simulink model "RW_1_testmode"  (R2018a)
settings: Solver=ode4  StartTime=0  StopTime=1000  FixedStep=ConfParam.confOrbit.dt  RelTol=1e-3
undefined symbols (not defined in the file): ConfParam, import_orbit, RWS, Subsystem
libraries: ComputeNorm3D x5, simulink x4, sharedtransform x2, Command x1, Date x1, KepOrbit x1, Estimator x1, BdotController x1, RWS_1W_PDcontroller x1, IGRF x1, SunEphemeris_MathWorks x1, MTB x1
settings Model: Creator=Cédric  LastModifiedBy=Cédric
settings DataIOCC: SaveTime=off
settings DebuggingCC: MultiTaskRateTransMsg=warning

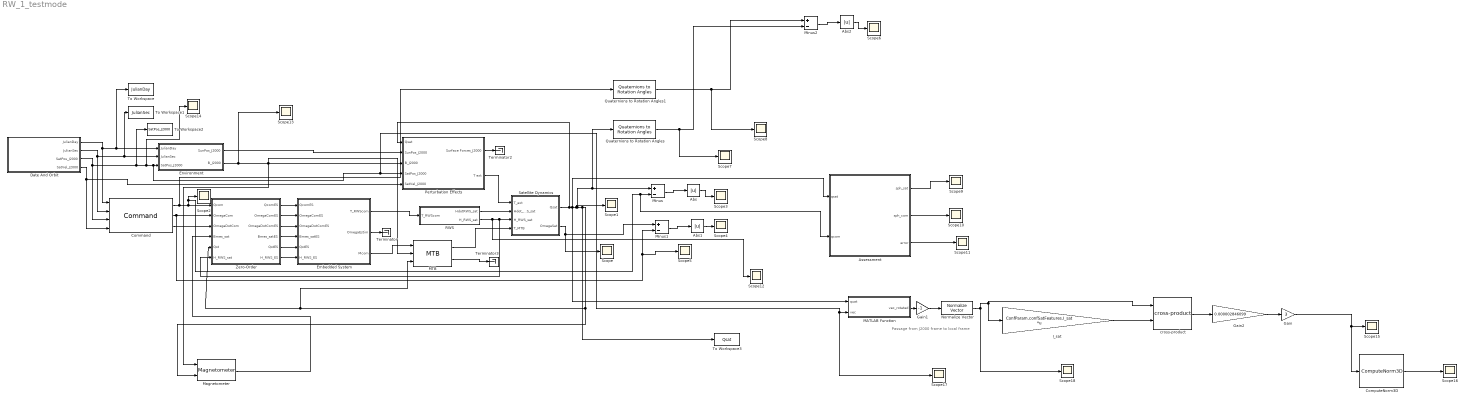
== system RW_1_testmode ==
  note: Passage from J2000 frame to local frame
  Abs : Abs
  Abs1 : Abs
  Abs2 : Abs
  Assessment : Subsystem
  Command : Command/Command
  ComputeNorm3D : ComputeNorm3D/ComputeNorm3D
  Date And Orbit : Subsystem
  Embedded System : Subsystem
  Environment : Subsystem
  Gain : Gain  Gain=3
  Gain1 : Gain  Gain=-1
  Gain2 : Gain  Gain=0.000002846099
  I_sat : Gain  Gain=ConfParam.confSatFeatures.I_sat  Multiplication=Matrix(K*u)
  MATLAB Function : MATLAB Function  TreatAsAtomicUnit=on
  MTB : MTB/MTB
  Magnetometer : Magnetometer/Magnetometer
  Minus : Sum  Inputs=+-
  Minus1 : Sum  Inputs=+-
  Minus2 : Sum  Inputs=+-
  Normalize Vector : vrlib/Utilities/Normalize Vector  maxzero=0
      settings: SourceProductName=Simulink 3D Animation  SourceProductBaseCode=VR
  Perturbation Effects : Subsystem
  Quaternions to Rotation Angles : sharedtransform/Quaternions to Rotation Angles  rotationOrder=ZYX  aMode=aMode
      settings: SourceProductBaseCode=AE
  Quaternions to Rotation Angles1 : sharedtransform/Quaternions to Rotation Angles  rotationOrder=ZYX  aMode=aMode
      settings: SourceProductBaseCode=AE
  RWS : Subsystem  AncestorBlock=RWS/RWS
  Satellite Dynamics : Subsystem  AncestorBlock=SatDyn/Satellite Dynamics
  Scope{,1..18} (19 alike) : Scope
  Terminator : Terminator
  Terminator2 : Terminator
  Terminator3 : Terminator
  To Workspace : ToWorkspace  VariableName=JulianDay  SampleTime=-1
  To Workspace1 : ToWorkspace  VariableName=JulianSec  SampleTime=-1
  To Workspace2 : ToWorkspace  VariableName=SatPos_J2000  SampleTime=-1
  To Workspace3 : ToWorkspace  VariableName=Qsat  SampleTime=-1
  Zero-Order : Subsystem
  cross-product : CrossProd/cross-product
  wires:
  Date And Orbit/1(JulianDay) -> To Workspace/1, Environment/1(JulianDay), Command/1
  Date And Orbit/2(JulianSec) -> To Workspace1/1, Environment/2(JulianSec), Command/2
  Date And Orbit/3(SatPos_J2000) -> To Workspace2/1, Scope14/1, Scope17/1, MATLAB Function/2(vec), Perturbation Effects/4(SatPos_J2000), Environment/3(SatPos_J2000), Command/3
  Date And Orbit/4(SatVel_J2000) -> Perturbation Effects/5(SatVel_J2000), Command/4
  Environment/1(SunPos_J2000) -> Perturbation Effects/2(SunPos_J2000)
  Environment/2(B_J2000) -> Scope13/1, Perturbation Effects/3(B_J2000), Magnetometer/1, MTB/2
  Command/1 -> Quaternions to Rotation Angles1/1, Assessment/2(qcom), Minus/2, Scope2/1, Zero-Order/1(Qcom)
  Command/2 -> Scope5/1, Minus1/2, Zero-Order/2(OmegaCom)
  Command/3 -> Zero-Order/3(OmegaDotCom)
  Zero-Order/1(QcomES) -> Embedded System/1(QcomES)
  Zero-Order/2(OmegaComES) -> Embedded System/2(OmegaComES)
  Zero-Order/3(OmegaDotComES) -> Embedded System/3(OmegaDotComES)
  Zero-Order/4(Bmes_satES) -> Embedded System/4(Bmes_satES)
  Zero-Order/5(QstES) -> Embedded System/5(QstES)
  Zero-Order/6(H_RWS_ES) -> Embedded System/6(H_RWS_ES)
  Embedded System/3(Mcom) -> MTB/1
  MTB/1 -> Satellite Dynamics/4(T_MTB)
  Magnetometer/1 -> Zero-Order/4(Bmes_sat)
  Embedded System/2(OmegaEstim) -> Terminator/1
  Satellite Dynamics/2(OmegaSat) -> Minus1/1, Scope/1
  Perturbation Effects/1(Surface Forces_J2000) -> Terminator2/1
  Minus/1 -> Abs/1
  Abs/1 -> Scope3/1
  Minus1/1 -> Abs1/1
  Abs1/1 -> Scope4/1
  Abs2/1 -> Scope6/1
  Minus2/1 -> Abs2/1
  Quaternions to Rotation Angles1/1 -> Scope8/1, Minus2/1
  Quaternions to Rotation Angles/1 -> Scope7/1, Minus2/2
  MTB/2 -> Terminator3/1
  RWS/2(H_RWS_sat) -> Scope12/1, Satellite Dynamics/3(H_RWS_sat), Zero-Order/6(H_RWS_sat)
  Embedded System/1(T_RWScom) -> RWS/1(T_RWScom)
  Perturbation Effects/2(T ext) -> Satellite Dynamics/1(T_ext)
  RWS/1(HdotRWS_sat) -> Satellite Dynamics/2(Hdot_RWS_sat)
  Gain2/1 -> Gain/1
  Gain/1 -> ComputeNorm3D/1, Scope15/1
  cross-product/1 -> Gain2/1
  I_sat/1 -> cross-product/2
  MATLAB Function/1(vec_rotated) -> Gain1/1
  ComputeNorm3D/1 -> Scope16/1
  Assessment/3(error) -> Scope11/1
  Assessment/2(sph_com) -> Scope10/1
  Assessment/1(sph_sat) -> Scope9/1
  Satellite Dynamics/1(Qsat) -> Perturbation Effects/1(Qsat), MATLAB Function/1(quat), Assessment/1(qsat), Scope1/1, Quaternions to Rotation Angles/1, Minus/1, To Workspace3/1, MTB/3, Zero-Order/5(Qst), Magnetometer/2
  Gain1/1 -> Normalize Vector/1
  Normalize Vector/1 -> I_sat/1, cross-product/1, Scope18/1

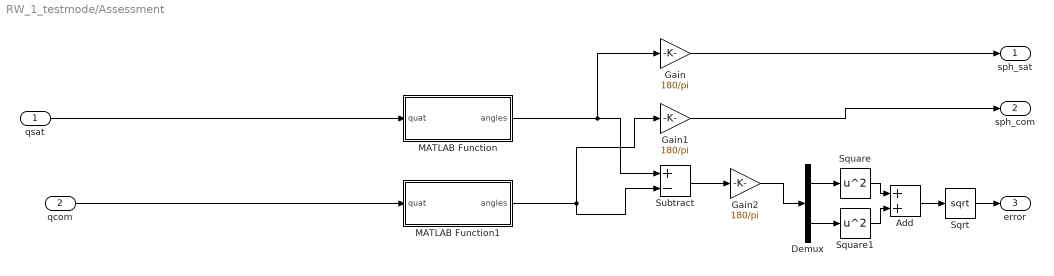
== system RW_1_testmode/Assessment ==
  qsat : Inport
  qcom : Inport  Port=2
  Add : Sum
  Demux : Demux  Outputs=2
  Gain : Gain  Gain=180/pi
  Gain1 : Gain  Gain=180/pi
  Gain2 : Gain  Gain=180/pi
  MATLAB Function : MATLAB Function  TreatAsAtomicUnit=on
  MATLAB Function1 : MATLAB Function  TreatAsAtomicUnit=on
  Sqrt : Sqrt  SaturateOnIntegerOverflow=on
  Square : Math  Operator=square  SaturateOnIntegerOverflow=on
  Square1 : Math  Operator=square  SaturateOnIntegerOverflow=on
  Subtract : Sum  Inputs=+-
  sph_sat : Outport
  sph_com : Outport  Port=2
  error : Outport  Port=3
  wires:
  MATLAB Function1/1(angles) -> Subtract/2, Gain1/1
  MATLAB Function/1(angles) -> Gain/1, Subtract/1
  Subtract/1 -> Gain2/1
  qsat/1 -> MATLAB Function/1(quat)
  Gain/1 -> sph_sat/1
  Gain1/1 -> sph_com/1
  Gain2/1 -> Demux/1
  Demux/1 -> Square/1
  Demux/2 -> Square1/1
  Square/1 -> Add/1
  Square1/1 -> Add/2
  Add/1 -> Sqrt/1
  Sqrt/1 -> error/1
  qcom/1 -> MATLAB Function1/1(quat)

== system RW_1_testmode/Date And Orbit ==
  Clock : Clock
  Current Simulation Date : Date/Current Simulation Date
  Orbit : KepOrbit/Keplerian Orbit
  Pierre's orbit : Subsystem  Commented=on  AncestorBlock=import_orbit/Subsystem
  JulianDay : Outport
  JulianSec : Outport  Port=2
  SatPos_J2000 : Outport  Port=3
  SatVel_J2000 : Outport  Port=4
  wires:
  Current Simulation Date/1 -> JulianDay/1
  Current Simulation Date/2 -> JulianSec/1
  Clock/1 -> Current Simulation Date/1
  Orbit/2 -> SatVel_J2000/1
  Orbit/1 -> SatPos_J2000/1

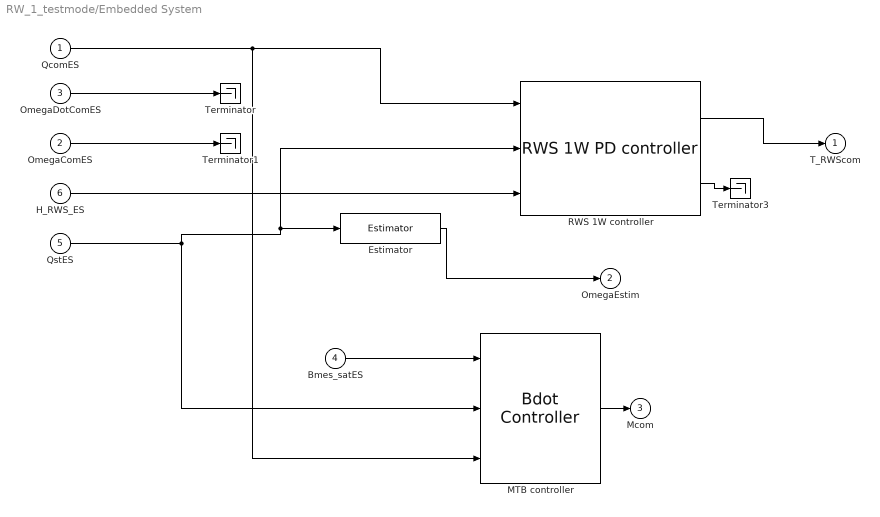
== system RW_1_testmode/Embedded System ==
  QcomES : Inport
  OmegaComES : Inport  Port=2
  OmegaDotComES : Inport  Port=3
  Bmes_satES : Inport  Port=4
  QstES : Inport  Port=5
  H_RWS_ES : Inport  Port=6
  Estimator : Estimator/Estimator
  MTB controller : BdotController/Bdot Controller
  RWS 1W controller : RWS_1W_PDcontroller/RWS 1W PD controller
  Terminator : Terminator
  Terminator1 : Terminator
  Terminator3 : Terminator
  T_RWScom : Outport
  OmegaEstim : Outport  Port=2
  Mcom : Outport  Port=3
  wires:
  QstES/1 -> MTB controller/2, RWS 1W controller/2, Estimator/1
  Estimator/1 -> OmegaEstim/1
  Bmes_satES/1 -> MTB controller/1
  MTB controller/1 -> Mcom/1
  QcomES/1 -> MTB controller/3, RWS 1W controller/1
  H_RWS_ES/1 -> RWS 1W controller/3
  OmegaComES/1 -> Terminator1/1
  OmegaDotComES/1 -> Terminator/1
  RWS 1W controller/1 -> T_RWScom/1
  RWS 1W controller/2 -> Terminator3/1

== system RW_1_testmode/Environment ==
  JulianDay : Inport
  JulianSec : Inport  Port=2
  SatPos_J2000 : Inport  Port=3
  B J2000 : IGRF/IGRF in the J2000 frame
  Sun Ephemeris J2000 : SunEphemeris_MathWorks/Sun Ephemeris J2000
  SunPos_J2000 : Outport
  B_J2000 : Outport  Port=2
  wires:
  Sun Ephemeris J2000/1 -> SunPos_J2000/1
  JulianDay/1 -> Sun Ephemeris J2000/1, B J2000/1
  JulianSec/1 -> Sun Ephemeris J2000/2, B J2000/2
  SatPos_J2000/1 -> B J2000/3
  B J2000/1 -> B_J2000/1

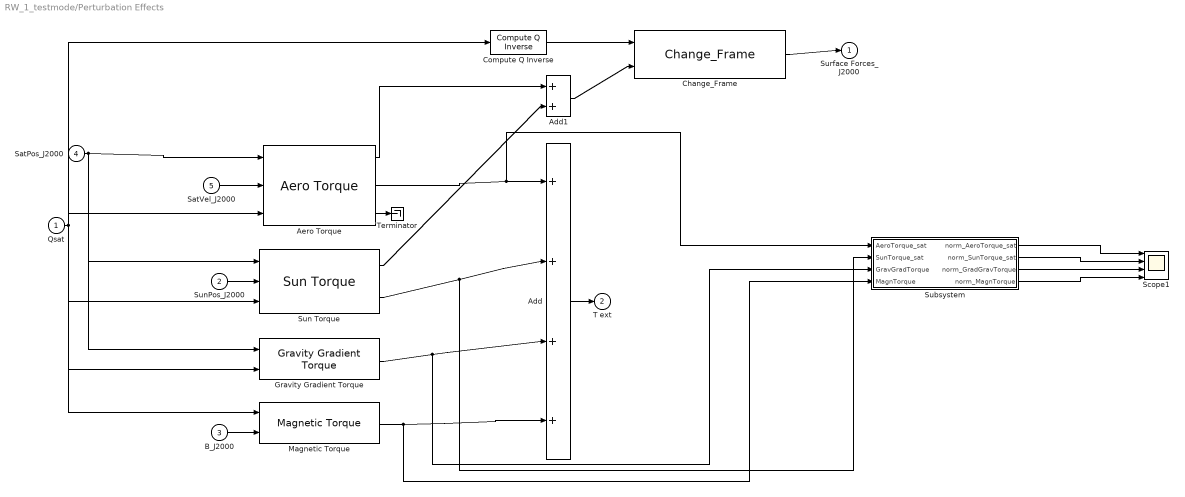
== system RW_1_testmode/Perturbation Effects ==
  Qsat : Inport
  SunPos_J2000 : Inport  Port=2
  B_J2000 : Inport  Port=3
  SatPos_J2000 : Inport  Port=4
  SatVel_J2000 : Inport  Port=5
  Add : Sum  Inputs=++++
  Add1 : Sum
  Aero Torque : AeroTorqueA/Aero Torque
  Change_Frame : ChangeFrame/Change_Frame
  Compute Q Inverse : Qinverse/Compute Q Inverse
  Gravity Gradient Torque : GravGradTorque/Gravity Gradient Torque
  Magnetic Torque : MagnTorque/Magnetic Torque
  Scope1 : Scope  NumInputPorts=4
  Subsystem : Subsystem
  Sun Torque : SunTorqueA/Sun Torque
  Terminator : Terminator
  Surface Forces_J2000 : Outport
  T ext : Outport  Port=2
  wires:
  Compute Q Inverse/1 -> Change_Frame/1
  Change_Frame/1 -> Surface Forces_J2000/1
  Qsat/1 -> Compute Q Inverse/1, Gravity Gradient Torque/2, Sun Torque/3, Magnetic Torque/1, Aero Torque/3
  SunPos_J2000/1 -> Sun Torque/2
  B_J2000/1 -> Magnetic Torque/2
  SatPos_J2000/1 -> Sun Torque/1, Gravity Gradient Torque/1, Aero Torque/1
  SatVel_J2000/1 -> Aero Torque/2
  Aero Torque/3 -> Terminator/1
  Add1/1 -> Change_Frame/2
  Aero Torque/1 -> Add1/1
  Sun Torque/1 -> Add1/2
  Add/1 -> T ext/1
  Aero Torque/2 -> Subsystem/1(AeroTorque_sat), Add/1
  Sun Torque/2 -> Subsystem/2(SunTorque_sat), Add/2
  Gravity Gradient Torque/1 -> Subsystem/3(GravGradTorque), Add/3
  Magnetic Torque/1 -> Subsystem/4(MagnTorque), Add/4
  Subsystem/1(norm_AeroTorque_sat) -> Scope1/1
  Subsystem/2(norm_SunTorque_sat) -> Scope1/2
  Subsystem/3(norm_GradGravTorque) -> Scope1/3
  Subsystem/4(norm_MagnTorque) -> Scope1/4

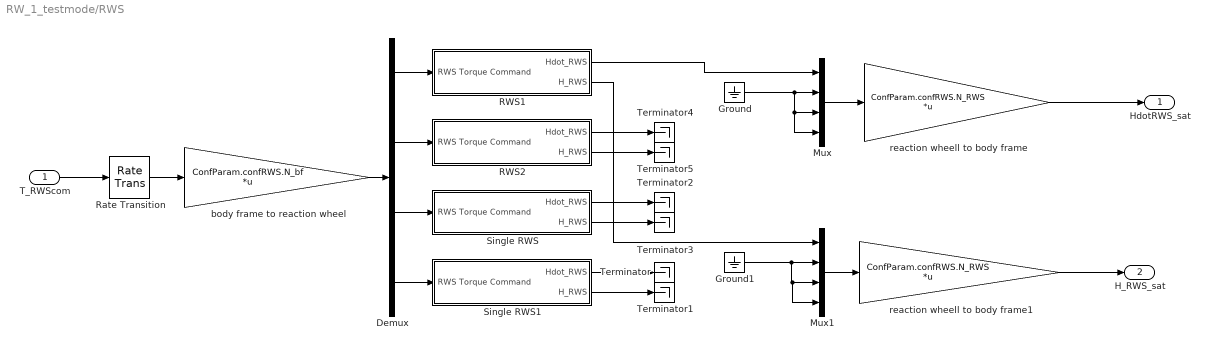
== system RW_1_testmode/RWS ==
  T_RWScom : Inport
  Demux : Demux
  Ground : Ground
  Ground1 : Ground
  Mux : Mux
  Mux1 : Mux
  RWS1 : Subsystem  AncestorBlock=SingleRWS/Single RWS
  RWS2 : Subsystem
  Rate Transition : RateTransition  InitialCondition=[0;0;0]  OutPortSampleTime=ConfParam.confOrbit.dt
  Single RWS : Subsystem
  Single RWS1 : Subsystem
  Terminator{,1..5} (6 alike) : Terminator
  body frame to reaction wheel : Gain  Gain=ConfParam.confRWS.N_bf  Multiplication=Matrix(K*u)
  reaction wheell to body frame : Gain  Gain=ConfParam.confRWS.N_RWS  Multiplication=Matrix(K*u)
  reaction wheell to body frame1 : Gain  Gain=ConfParam.confRWS.N_RWS  Multiplication=Matrix(K*u)
  HdotRWS_sat : Outport
  H_RWS_sat : Outport  Port=2
  wires:
  Ground1/1 -> Mux1/2, Mux1/3, Mux1/4
  Ground/1 -> Mux/2, Mux/3, Mux/4
  RWS2/2(H_RWS) -> Terminator5/1
  RWS2/1(Hdot_RWS) -> Terminator4/1
  Single RWS/2(H_RWS) -> Terminator3/1
  Single RWS/1(Hdot_RWS) -> Terminator2/1
  Single RWS1/2(H_RWS) -> Terminator1/1
  Single RWS1/1(Hdot_RWS) -> Terminator/1
  Mux1/1 -> reaction wheell to body frame1/1
  Demux/2 -> RWS2/1(RWS Torque Command)
  Demux/4 -> Single RWS1/1(RWS Torque Command)
  Demux/3 -> Single RWS/1(RWS Torque Command)
  RWS1/1(Hdot_RWS) -> Mux/1
  reaction wheell to body frame/1 -> HdotRWS_sat/1
  reaction wheell to body frame1/1 -> H_RWS_sat/1
  RWS1/2(H_RWS) -> Mux1/1
  Mux/1 -> reaction wheell to body frame/1
  Demux/1 -> RWS1/1(RWS Torque Command)
  body frame to reaction wheel/1 -> Demux/1
  T_RWScom/1 -> Rate Transition/1
  Rate Transition/1 -> body frame to reaction wheel/1

== system RW_1_testmode/Satellite Dynamics ==
  T_ext : Inport
  Hdot_RWS_sat : Inport  Port=2
  H_RWS_sat : Inport  Port=3
  T_MTB : Inport  Port=4
  Compute Omega Sat : Subsystem
  Constant : Constant  Value=0
  Gain : Gain  Gain=1/2
  Integrator : Integrator  InitialCondition=ConfParam.confSatDyn.InitQsat
  Mux : Mux  Inputs=2
  QuatProd : Subsystem  TreatAsAtomicUnit=on
      settings: RTWFcnNameOpts=Use subsystem name  RTWFileNameOpts=Use subsystem name
  Qsat : Outport
  OmegaSat : Outport  Port=2
  wires:
  H_RWS_sat/1 -> Compute Omega Sat/3(H_RWS_sat)
  QuatProd/1("q\"") -> Gain/1
  T_MTB/1 -> Compute Omega Sat/4(T_MTB)
  Constant/1 -> Mux/1
  Hdot_RWS_sat/1 -> Compute Omega Sat/2(Hdot_RWS_sat)
  Gain/1 -> Integrator/1
  Integrator/1 -> QuatProd/1(q), Qsat/1
  Mux/1 -> QuatProd/2(q')
  Compute Omega Sat/1(OmegaSat) -> Mux/2, OmegaSat/1
  T_ext/1 -> Compute Omega Sat/1(T_ext)

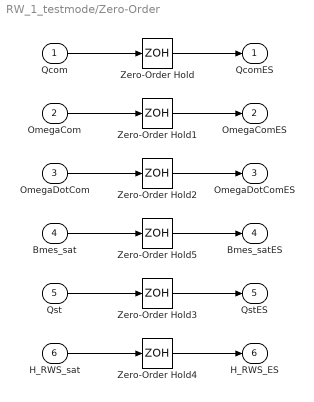
== system RW_1_testmode/Zero-Order ==
  Qcom : Inport
  OmegaCom : Inport  Port=2
  OmegaDotCom : Inport  Port=3
  Bmes_sat : Inport  Port=4
  Qst : Inport  Port=5
  H_RWS_sat : Inport  Port=6
  Zero-Order Hold{,1..5} (6 alike) : ZeroOrderHold  SampleTime=1/ConfParam.confES.frequency
  QcomES : Outport
  OmegaComES : Outport  Port=2
  OmegaDotComES : Outport  Port=3
  Bmes_satES : Outport  Port=4
  QstES : Outport  Port=5
  H_RWS_ES : Outport  Port=6
  wires:
  Qcom/1 -> Zero-Order Hold/1
  Zero-Order Hold/1 -> QcomES/1
  OmegaCom/1 -> Zero-Order Hold1/1
  Zero-Order Hold1/1 -> OmegaComES/1
  OmegaDotCom/1 -> Zero-Order Hold2/1
  Zero-Order Hold2/1 -> OmegaDotComES/1
  Qst/1 -> Zero-Order Hold3/1
  Zero-Order Hold3/1 -> QstES/1
  H_RWS_sat/1 -> Zero-Order Hold4/1
  Zero-Order Hold4/1 -> H_RWS_ES/1
  Bmes_sat/1 -> Zero-Order Hold5/1
  Zero-Order Hold5/1 -> Bmes_satES/1

== system RW_1_testmode/Date And Orbit/Pierre's orbit ==
  Demux : Demux  Outputs=6
  From File : FromFile  FileName=C:\Users\cedri\Documents\TOLOSAT\tolosat_adcs\pythondev\positions\timestamped_file.mat  SampleTime=1  ExtrapolationBeforeFirstDataPoint=Hold first value  InterpolationWithinTimeRange=Zero order hold  ExtrapolationAfterLastDataPoint=Hold last value
  Mux : Mux  Inputs=3
  Mux1 : Mux  Inputs=3
  Positions : Scope
  Velocities : Scope
  SatVel_J2000 : Outport
  SatPos_J2000 : Outport  Port=2
  wires:
  Demux/6 -> Mux1/3
  Mux1/1 -> Positions/1, SatPos_J2000/1
  Demux/4 -> Mux1/1
  From File/1 -> Demux/1
  Mux/1 -> Velocities/1, SatVel_J2000/1
  Demux/1 -> Mux/1
  Demux/2 -> Mux/2
  Demux/3 -> Mux/3
  Demux/5 -> Mux1/2

== system RW_1_testmode/Perturbation Effects/Subsystem ==
  AeroTorque_sat : Inport
  SunTorque_sat : Inport  Port=2
  GravGradTorque : Inport  Port=3
  MagnTorque : Inport  Port=4
  ComputeNorm3D{,1..3} (4 alike) : ComputeNorm3D/ComputeNorm3D
  norm_AeroTorque_sat : Outport
  norm_SunTorque_sat : Outport  Port=2
  norm_GradGravTorque : Outport  Port=3
  norm_MagnTorque : Outport  Port=4
  wires:
  GravGradTorque/1 -> ComputeNorm3D1/1
  ComputeNorm3D1/1 -> norm_GradGravTorque/1
  AeroTorque_sat/1 -> ComputeNorm3D/1
  MagnTorque/1 -> ComputeNorm3D3/1
  ComputeNorm3D2/1 -> norm_SunTorque_sat/1
  SunTorque_sat/1 -> ComputeNorm3D2/1
  ComputeNorm3D3/1 -> norm_MagnTorque/1
  ComputeNorm3D/1 -> norm_AeroTorque_sat/1

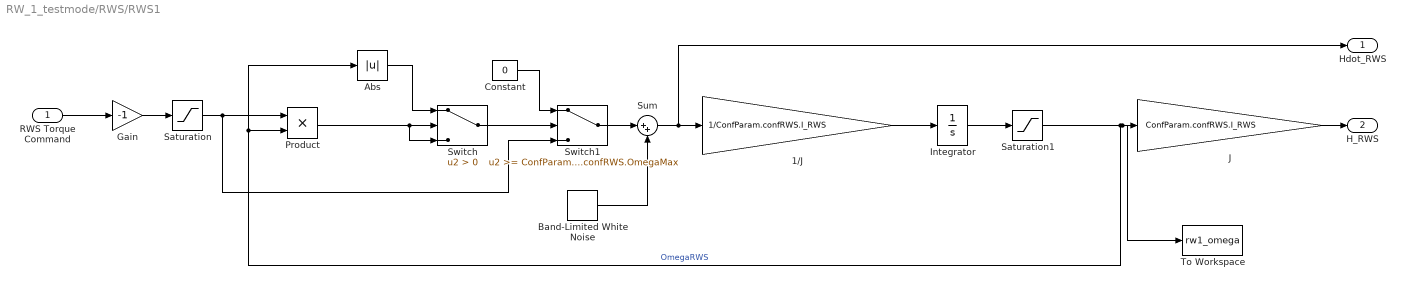
== system RW_1_testmode/RWS/RWS1 ==
  RWS Torque Command : Inport
  1/J : Gain  Gain=1/ConfParam.confRWS.I_RWS
  Abs : Abs
  Band-Limited White Noise : simulink/Sources/Band-Limited White Noise  Cov=ConfParam.confRWS.NoisePower  Ts=ConfParam.confOrbit.dt  seed=[23341]
  Constant : Constant  Value=0
  Gain : Gain  Gain=-1
  Integrator : Integrator  InitialCondition=ConfParam.confRWS.IntitOmegaRWS(1)
  J : Gain  Gain=ConfParam.confRWS.I_RWS
  Product : Product
  Saturation : Saturate  UpperLimit=ConfParam.confRWS.Tmax  LowerLimit=-ConfParam.confRWS.Tmax
  Saturation1 : Saturate  UpperLimit=ConfParam.confRWS.OmegaMax  LowerLimit=-ConfParam.confRWS.OmegaMax
  Sum : Sum  Inputs=|++
  Switch : Switch  Criteria=u2 > Threshold
  Switch1 : Switch  Threshold=ConfParam.confRWS.OmegaMax
  To Workspace : ToWorkspace  VariableName=rw1_omega  SampleTime=-1
  Hdot_RWS : Outport
  H_RWS : Outport  Port=2
  wires:
  Switch1/1 -> Sum/1
  Switch/1 -> Switch1/2
  Constant/1 -> Switch1/1
  RWS Torque Command/1 -> Gain/1
  Product/1 -> Switch/2, Switch/3
  Saturation/1 -> Product/1, Switch1/3
  Integrator/1 -> Saturation1/1
  Saturation1/1 -> To Workspace/1, J/1, Abs/1, Product/2  "OmegaRWS"
  Sum/1 -> Hdot_RWS/1, 1/J/1
  1/J/1 -> Integrator/1
  Abs/1 -> Switch/1
  J/1 -> H_RWS/1
  Band-Limited White Noise/1 -> Sum/2
  Gain/1 -> Saturation/1

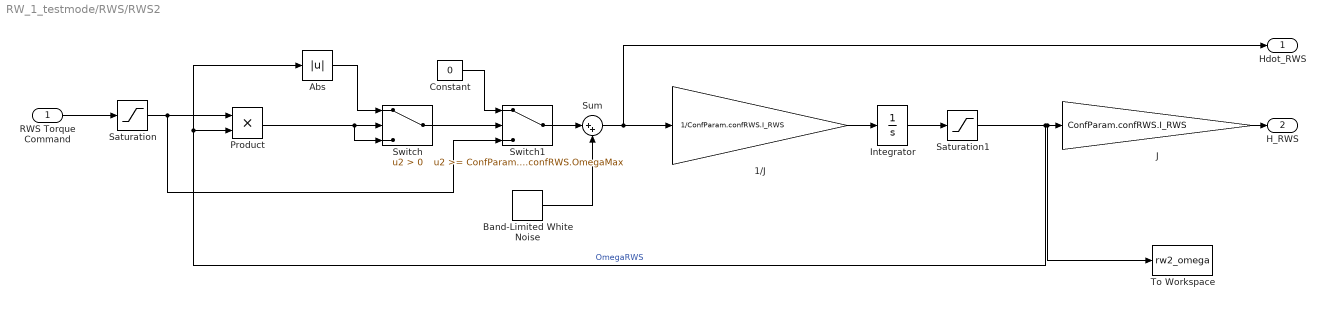
== system RW_1_testmode/RWS/RWS2 ==
  RWS Torque Command : Inport
  1/J : Gain  Gain=1/ConfParam.confRWS.I_RWS
  Abs : Abs
  Band-Limited White Noise : simulink/Sources/Band-Limited White Noise  Cov=ConfParam.confRWS.NoisePower  Ts=ConfParam.confOrbit.dt  seed=[23341]
  Constant : Constant  Value=0
  Integrator : Integrator  InitialCondition=ConfParam.confRWS.IntitOmegaRWS(2)
  J : Gain  Gain=ConfParam.confRWS.I_RWS
  Product : Product
  Saturation : Saturate  UpperLimit=ConfParam.confRWS.Tmax  LowerLimit=-ConfParam.confRWS.Tmax
  Saturation1 : Saturate  UpperLimit=ConfParam.confRWS.OmegaMax  LowerLimit=-ConfParam.confRWS.OmegaMax
  Sum : Sum  Inputs=|++
  Switch : Switch  Criteria=u2 > Threshold
  Switch1 : Switch  Threshold=ConfParam.confRWS.OmegaMax
  To Workspace : ToWorkspace  VariableName=rw2_omega  SampleTime=-1
  Hdot_RWS : Outport
  H_RWS : Outport  Port=2
  wires:
  Switch1/1 -> Sum/1
  Switch/1 -> Switch1/2
  Constant/1 -> Switch1/1
  RWS Torque Command/1 -> Saturation/1
  Product/1 -> Switch/2, Switch/3
  Saturation/1 -> Product/1, Switch1/3
  Integrator/1 -> Saturation1/1
  Saturation1/1 -> Abs/1, Product/2, To Workspace/1, J/1  "OmegaRWS"
  Sum/1 -> Hdot_RWS/1, 1/J/1
  1/J/1 -> Integrator/1
  Abs/1 -> Switch/1
  J/1 -> H_RWS/1
  Band-Limited White Noise/1 -> Sum/2

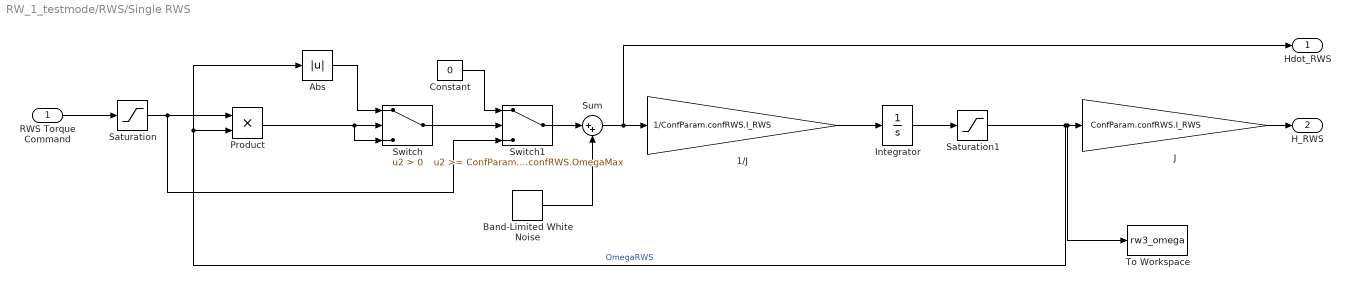
== system RW_1_testmode/RWS/Single RWS ==
  RWS Torque Command : Inport
  1/J : Gain  Gain=1/ConfParam.confRWS.I_RWS
  Abs : Abs
  Band-Limited White Noise : simulink/Sources/Band-Limited White Noise  Cov=ConfParam.confRWS.NoisePower  Ts=ConfParam.confOrbit.dt  seed=[23341]
  Constant : Constant  Value=0
  Integrator : Integrator  InitialCondition=ConfParam.confRWS.IntitOmegaRWS(3)
  J : Gain  Gain=ConfParam.confRWS.I_RWS
  Product : Product
  Saturation : Saturate  UpperLimit=ConfParam.confRWS.Tmax  LowerLimit=-ConfParam.confRWS.Tmax
  Saturation1 : Saturate  UpperLimit=ConfParam.confRWS.OmegaMax  LowerLimit=-ConfParam.confRWS.OmegaMax
  Sum : Sum  Inputs=|++
  Switch : Switch  Criteria=u2 > Threshold
  Switch1 : Switch  Threshold=ConfParam.confRWS.OmegaMax
  To Workspace : ToWorkspace  VariableName=rw3_omega  SampleTime=-1
  Hdot_RWS : Outport
  H_RWS : Outport  Port=2
  wires:
  Switch1/1 -> Sum/1
  Switch/1 -> Switch1/2
  Constant/1 -> Switch1/1
  RWS Torque Command/1 -> Saturation/1
  Product/1 -> Switch/2, Switch/3
  Saturation/1 -> Product/1, Switch1/3
  Integrator/1 -> Saturation1/1
  Saturation1/1 -> To Workspace/1, J/1, Abs/1, Product/2  "OmegaRWS"
  Sum/1 -> Hdot_RWS/1, 1/J/1
  1/J/1 -> Integrator/1
  Abs/1 -> Switch/1
  J/1 -> H_RWS/1
  Band-Limited White Noise/1 -> Sum/2

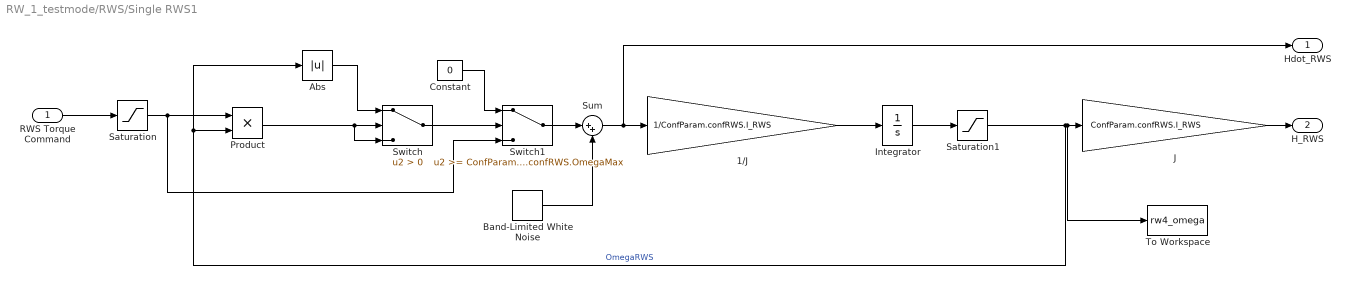
== system RW_1_testmode/RWS/Single RWS1 ==
  RWS Torque Command : Inport
  1/J : Gain  Gain=1/ConfParam.confRWS.I_RWS
  Abs : Abs
  Band-Limited White Noise : simulink/Sources/Band-Limited White Noise  Cov=ConfParam.confRWS.NoisePower  Ts=ConfParam.confOrbit.dt  seed=[23341]
  Constant : Constant  Value=0
  Integrator : Integrator  InitialCondition=ConfParam.confRWS.IntitOmegaRWS(4)
  J : Gain  Gain=ConfParam.confRWS.I_RWS
  Product : Product
  Saturation : Saturate  UpperLimit=ConfParam.confRWS.Tmax  LowerLimit=-ConfParam.confRWS.Tmax
  Saturation1 : Saturate  UpperLimit=ConfParam.confRWS.OmegaMax  LowerLimit=-ConfParam.confRWS.OmegaMax
  Sum : Sum  Inputs=|++
  Switch : Switch  Criteria=u2 > Threshold
  Switch1 : Switch  Threshold=ConfParam.confRWS.OmegaMax
  To Workspace : ToWorkspace  VariableName=rw4_omega  SampleTime=-1
  Hdot_RWS : Outport
  H_RWS : Outport  Port=2
  wires:
  Switch1/1 -> Sum/1
  Switch/1 -> Switch1/2
  Constant/1 -> Switch1/1
  RWS Torque Command/1 -> Saturation/1
  Product/1 -> Switch/2, Switch/3
  Saturation/1 -> Product/1, Switch1/3
  Integrator/1 -> Saturation1/1
  Saturation1/1 -> To Workspace/1, J/1, Abs/1, Product/2  "OmegaRWS"
  Sum/1 -> Hdot_RWS/1, 1/J/1
  1/J/1 -> Integrator/1
  Abs/1 -> Switch/1
  J/1 -> H_RWS/1
  Band-Limited White Noise/1 -> Sum/2

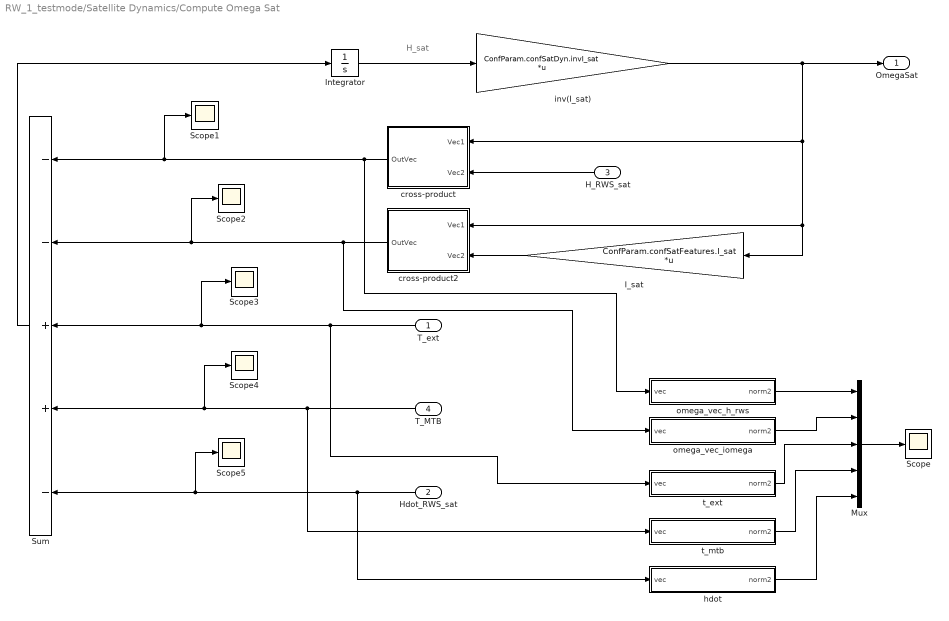
== system RW_1_testmode/Satellite Dynamics/Compute Omega Sat ==
  note: H_sat
  T_ext : Inport
  Hdot_RWS_sat : Inport  Port=2
  H_RWS_sat : Inport  Port=3
  T_MTB : Inport  Port=4
  I_sat : Gain  Gain=ConfParam.confSatFeatures.I_sat  Multiplication=Matrix(K*u)
  Integrator : Integrator  InitialCondition=ConfParam.confSatFeatures.I_sat*ConfParam.confSatDyn.InitOmega_sat
  Mux : Mux  Inputs=5
  Scope{,1..5} (6 alike) : Scope
  Sum : Sum  Inputs=--++-
  cross-product : Subsystem
  cross-product2 : Subsystem
  hdot : Subsystem
  inv(I_sat) : Gain  Gain=ConfParam.confSatDyn.invI_sat  Multiplication=Matrix(K*u)
  omega_vec_h_rws : Subsystem
  omega_vec_iomega : Subsystem
  t_ext : Subsystem
  t_mtb : Subsystem
  OmegaSat : Outport
  wires:
  Mux/1 -> Scope/1
  H_RWS_sat/1 -> cross-product/2(Vec2)
  I_sat/1 -> cross-product2/2(Vec2)
  T_ext/1 -> t_ext/1(vec), Scope3/1, Sum/3
  T_MTB/1 -> t_mtb/1(vec), Sum/4, Scope4/1
  Sum/1 -> Integrator/1
  inv(I_sat)/1 -> OmegaSat/1, I_sat/1, cross-product2/1(Vec1), cross-product/1(Vec1)
  Integrator/1 -> inv(I_sat)/1
  hdot/1(norm2) -> Mux/5
  t_mtb/1(norm2) -> Mux/4
  t_ext/1(norm2) -> Mux/3
  omega_vec_iomega/1(norm2) -> Mux/2
  omega_vec_h_rws/1(norm2) -> Mux/1
  cross-product2/1(OutVec) -> Scope2/1, Sum/2, omega_vec_iomega/1(vec)
  cross-product/1(OutVec) -> Scope1/1, Sum/1, omega_vec_h_rws/1(vec)
  Hdot_RWS_sat/1 -> Scope5/1, Sum/5, hdot/1(vec)

== system RW_1_testmode/Satellite Dynamics/QuatProd ==
  note: Quaternion product : q" = q.q'
  q : Inport  OutDataTypeStr=double  PortDimensions=4
  q' : Inport  Port=2  OutDataTypeStr=double  PortDimensions=4
  1,-2,-3,-4 : Gain  Gain=[1 0 0 0;0 -1 0 0;0 0 -1 0;0 0 0 -1]  Multiplication=Matrix(K*u) (u vector)  SaturateOnIntegerOverflow=on  OutDataTypeStr=Inherit: Same as input  ParamDataTypeStr=Inherit: Same as input
  2,1,4,-3 : Gain  Gain=[0 1 0 0 ; 1 0 0 0 ; 0 0 0 1 ; 0 0 -1 0]  Multiplication=Matrix(K*u) (u vector)  SaturateOnIntegerOverflow=on  OutDataTypeStr=Inherit: Same as input  ParamDataTypeStr=Inherit: Same as input
  3,-4,1,2 : Gain  Gain=[0 0 1 0 ; 0 0 0 -1 ; 1 0 0 0 ; 0 1 0 0]  Multiplication=Matrix(K*u) (u vector)  SaturateOnIntegerOverflow=on  OutDataTypeStr=Inherit: Same as input  ParamDataTypeStr=Inherit: Same as input
  4,3,-2,1 : Gain  Gain=[0 0 0 1;0 0 1 0 ; 0 -1 0 0 ; 1 0 0 0]  Multiplication=Matrix(K*u) (u vector)  SaturateOnIntegerOverflow=on  OutDataTypeStr=Inherit: Same as input  ParamDataTypeStr=Inherit: Same as input
  Dot Product{,1..3} (4 alike) : DotProduct  InputSameDT=on  OutDataTypeStr=Inherit: Inherit via internal rule
  Mux : Mux
  "q\"" : Outport  OutDataTypeStr=double  PortDimensions=4  InitialOutput=0
  wires:
  Mux/1 -> "q\""/1
  Dot Product3/1 -> Mux/4
  Dot Product2/1 -> Mux/3
  Dot Product1/1 -> Mux/2
  Dot Product/1 -> Mux/1
  q/1 -> Dot Product3/1, Dot Product2/1, Dot Product1/1, Dot Product/1
  4,3,-2,1/1 -> Dot Product3/2
  3,-4,1,2/1 -> Dot Product2/2
  2,1,4,-3/1 -> Dot Product1/2
  1,-2,-3,-4/1 -> Dot Product/2
  q'/1 -> 2,1,4,-3/1, 1,-2,-3,-4/1, 4,3,-2,1/1, 3,-4,1,2/1

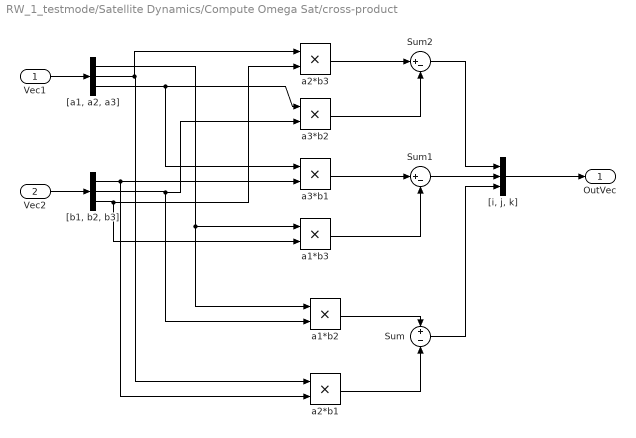
== system RW_1_testmode/Satellite Dynamics/Compute Omega Sat/cross-product ==
  Vec1 : Inport
  Vec2 : Inport  Port=2
  Sum : Sum  Inputs=+-
  Sum1 : Sum  Inputs=|+-
  Sum2 : Sum  Inputs=|+-
  "[a1, a2, a3]" : Demux  Outputs=3
  "[b1, b2, b3]" : Demux  Outputs=3
  "[i, j, k]" : Mux  Inputs=3
  a1*b2 : Product
  a1*b3 : Product
  a2*b1 : Product
  a2*b3 : Product
  a3*b1 : Product
  a3*b2 : Product
  OutVec : Outport
  wires:
  Sum1/1 -> "[i, j, k]"/2
  Sum2/1 -> "[i, j, k]"/1
  Sum/1 -> "[i, j, k]"/3
  a3*b2/1 -> Sum2/2
  "[i, j, k]"/1 -> OutVec/1
  a1*b3/1 -> Sum1/2
  "[b1, b2, b3]"/3 -> a1*b3/2, a2*b3/2
  a2*b3/1 -> Sum2/1
  "[a1, a2, a3]"/3 -> a3*b2/1, a3*b1/1
  a3*b1/1 -> Sum1/1
  a1*b2/1 -> Sum/1
  "[b1, b2, b3]"/2 -> a1*b2/2, a3*b2/2
  Vec1/1 -> "[a1, a2, a3]"/1
  "[a1, a2, a3]"/1 -> a1*b2/1, a1*b3/1
  Vec2/1 -> "[b1, b2, b3]"/1
  "[a1, a2, a3]"/2 -> a2*b1/1, a2*b3/1
  "[b1, b2, b3]"/1 -> a2*b1/2, a3*b1/2
  a2*b1/1 -> Sum/2

== system RW_1_testmode/Satellite Dynamics/Compute Omega Sat/cross-product2 ==
  Vec1 : Inport
  Vec2 : Inport  Port=2
  Sum : Sum  Inputs=+-
  Sum1 : Sum  Inputs=|+-
  Sum2 : Sum  Inputs=|+-
  "[a1, a2, a3]" : Demux  Outputs=3
  "[b1, b2, b3]" : Demux  Outputs=3
  "[i, j, k]" : Mux  Inputs=3
  a1*b2 : Product
  a1*b3 : Product
  a2*b1 : Product
  a2*b3 : Product
  a3*b1 : Product
  a3*b2 : Product
  OutVec : Outport
  wires:
  Sum1/1 -> "[i, j, k]"/2
  Sum2/1 -> "[i, j, k]"/1
  Sum/1 -> "[i, j, k]"/3
  a3*b2/1 -> Sum2/2
  "[i, j, k]"/1 -> OutVec/1
  a1*b3/1 -> Sum1/2
  "[b1, b2, b3]"/3 -> a1*b3/2, a2*b3/2
  a2*b3/1 -> Sum2/1
  "[a1, a2, a3]"/3 -> a3*b2/1, a3*b1/1
  a3*b1/1 -> Sum1/1
  a1*b2/1 -> Sum/1
  "[b1, b2, b3]"/2 -> a1*b2/2, a3*b2/2
  Vec1/1 -> "[a1, a2, a3]"/1
  "[a1, a2, a3]"/1 -> a1*b2/1, a1*b3/1
  Vec2/1 -> "[b1, b2, b3]"/1
  "[a1, a2, a3]"/2 -> a2*b1/1, a2*b3/1
  "[b1, b2, b3]"/1 -> a2*b1/2, a3*b1/2
  a2*b1/1 -> Sum/2

== system RW_1_testmode/Satellite Dynamics/Compute Omega Sat/hdot ==
  vec : Inport
  Demux : Demux  Outputs=3
  Sqrt : Sqrt  SaturateOnIntegerOverflow=on
  Square : Math  Operator=square  SaturateOnIntegerOverflow=on
  Square1 : Math  Operator=square  SaturateOnIntegerOverflow=on
  Square2 : Math  Operator=square  SaturateOnIntegerOverflow=on
  Sum1 : Sum  Inputs=3
  norm2 : Outport
  wires:
  vec/1 -> Demux/1
  Sqrt/1 -> norm2/1
  Demux/2 -> Square1/1
  Square/1 -> Sum1/1
  Demux/3 -> Square2/1
  Square2/1 -> Sum1/3
  Square1/1 -> Sum1/2
  Demux/1 -> Square/1
  Sum1/1 -> Sqrt/1

== system RW_1_testmode/Satellite Dynamics/Compute Omega Sat/omega_vec_h_rws ==
  vec : Inport
  Demux : Demux  Outputs=3
  Sqrt : Sqrt  SaturateOnIntegerOverflow=on
  Square : Math  Operator=square  SaturateOnIntegerOverflow=on
  Square1 : Math  Operator=square  SaturateOnIntegerOverflow=on
  Square2 : Math  Operator=square  SaturateOnIntegerOverflow=on
  Sum1 : Sum  Inputs=3
  norm2 : Outport
  wires:
  vec/1 -> Demux/1
  Sqrt/1 -> norm2/1
  Demux/2 -> Square1/1
  Square/1 -> Sum1/1
  Demux/3 -> Square2/1
  Square2/1 -> Sum1/3
  Square1/1 -> Sum1/2
  Demux/1 -> Square/1
  Sum1/1 -> Sqrt/1

== system RW_1_testmode/Satellite Dynamics/Compute Omega Sat/omega_vec_iomega ==
  vec : Inport
  Demux : Demux  Outputs=3
  Sqrt : Sqrt  SaturateOnIntegerOverflow=on
  Square : Math  Operator=square  SaturateOnIntegerOverflow=on
  Square1 : Math  Operator=square  SaturateOnIntegerOverflow=on
  Square2 : Math  Operator=square  SaturateOnIntegerOverflow=on
  Sum1 : Sum  Inputs=3
  norm2 : Outport
  wires:
  vec/1 -> Demux/1
  Sqrt/1 -> norm2/1
  Demux/2 -> Square1/1
  Square/1 -> Sum1/1
  Demux/3 -> Square2/1
  Square2/1 -> Sum1/3
  Square1/1 -> Sum1/2
  Demux/1 -> Square/1
  Sum1/1 -> Sqrt/1

== system RW_1_testmode/Satellite Dynamics/Compute Omega Sat/t_ext ==
  vec : Inport
  Demux : Demux  Outputs=3
  Sqrt : Sqrt  SaturateOnIntegerOverflow=on
  Square : Math  Operator=square  SaturateOnIntegerOverflow=on
  Square1 : Math  Operator=square  SaturateOnIntegerOverflow=on
  Square2 : Math  Operator=square  SaturateOnIntegerOverflow=on
  Sum1 : Sum  Inputs=3
  norm2 : Outport
  wires:
  vec/1 -> Demux/1
  Sqrt/1 -> norm2/1
  Demux/2 -> Square1/1
  Square/1 -> Sum1/1
  Demux/3 -> Square2/1
  Square2/1 -> Sum1/3
  Square1/1 -> Sum1/2
  Demux/1 -> Square/1
  Sum1/1 -> Sqrt/1

== system RW_1_testmode/Satellite Dynamics/Compute Omega Sat/t_mtb ==
  vec : Inport
  Demux : Demux  Outputs=3
  Sqrt : Sqrt  SaturateOnIntegerOverflow=on
  Square : Math  Operator=square  SaturateOnIntegerOverflow=on
  Square1 : Math  Operator=square  SaturateOnIntegerOverflow=on
  Square2 : Math  Operator=square  SaturateOnIntegerOverflow=on
  Sum1 : Sum  Inputs=3
  norm2 : Outport
  wires:
  vec/1 -> Demux/1
  Sqrt/1 -> norm2/1
  Demux/2 -> Square1/1
  Square/1 -> Sum1/1
  Demux/3 -> Square2/1
  Square2/1 -> Sum1/3
  Square1/1 -> Sum1/2
  Demux/1 -> Square/1
  Sum1/1 -> Sqrt/1

== matlab function RW_1_testmode/Assessment/MATLAB Function1 ==
  data: quat input; angles output
function angles = extract_sph_angles(quat)

%%% extracts theta and phi from quaternion qsat
%%% here we consider the angles for the z-axis (0 0 1)
%%% but it can be changed to any other axis if necessary.

q0 = quat(1);
q1 = quat(2);
q2 = quat(3);
q3 = quat(4);
P = [2*(q0^2 + q1^2)-1 2*(q1*q2 - q0*q3) 2*(q1*q3 + q2*q0);
     2*(q1*q2 + q0*q3) 2*(q0^2 + q2^2)-1 2*(q2*q3 - q1*q0);
     2*(q1*q3 - q2*q0) 2*(q2*q3 + q1*q0) 2*(q0^2 + q3^2)-1];
prod = P*[0; 0; 1];
x = prod(1);
y = prod(2);
z = prod(3);
[phi, theta, r] = cart2sph(x, y, z);

angles = [theta; phi];

== matlab function RW_1_testmode/Assessment/MATLAB Function ==
  data: quat input; angles output
function angles = extract_sph_angles(quat)

%%% extracts theta and phi from quaternion qsat
%%% here we consider the angles for the z-axis (0 0 1)
%%% but it can be changed to any other axis if necessary.

q0 = quat(1);
q1 = quat(2);
q2 = quat(3);
q3 = quat(4);
P = [2*(q0^2 + q1^2)-1 2*(q1*q2 - q0*q3) 2*(q1*q3 + q2*q0);
     2*(q1*q2 + q0*q3) 2*(q0^2 + q2^2)-1 2*(q2*q3 - q1*q0);
     2*(q1*q3 - q2*q0) 2*(q2*q3 + q1*q0) 2*(q0^2 + q3^2)-1];
prod = P*[0; 0; 1];
x = prod(1);
y = prod(2);
z = prod(3);
[phi, theta, r] = cart2sph(x, y, z);

angles = [theta; phi];

== matlab function RW_1_testmode/MATLAB Function ==
  data: quat input; vec_rotated output; vec input
function vec_rotated = quat2rot_dot(quat, vec)

%%% returns rotation matrix from quaternion quat

q0 = quat(1);
q1 = quat(2);
q2 = quat(3);
q3 = quat(4);
P = [2*(q0^2 + q1^2)-1 2*(q1*q2 - q0*q3) 2*(q1*q3 + q2*q0);
     2*(q1*q2 + q0*q3) 2*(q0^2 + q2^2)-1 2*(q2*q3 - q1*q0);
     2*(q1*q3 - q2*q0) 2*(q2*q3 + q1*q0) 2*(q0^2 + q3^2)-1];
vec_rotated = P*vec;
